simulink model "FCC_2021_JEVG"  (R2021a)
settings: Solver=VariableStepAuto  StartTime=0.0  StopTime=10  RelTol=1e-3
libraries: fl_lib x8, nesl_utility x3
settings Model: Creator=mluser  LastModifiedBy=user
settings DebuggingCC: UnconnectedInputMsg=none  UnconnectedOutputMsg=none  UnconnectedLineMsg=none
settings ModelReferenceCC: EnableRefExpFcnMdlSchedulingChecks=off
settings RTWCC: Description=Generic Real-Time Target  DLArmComputeVersion=20.02.1

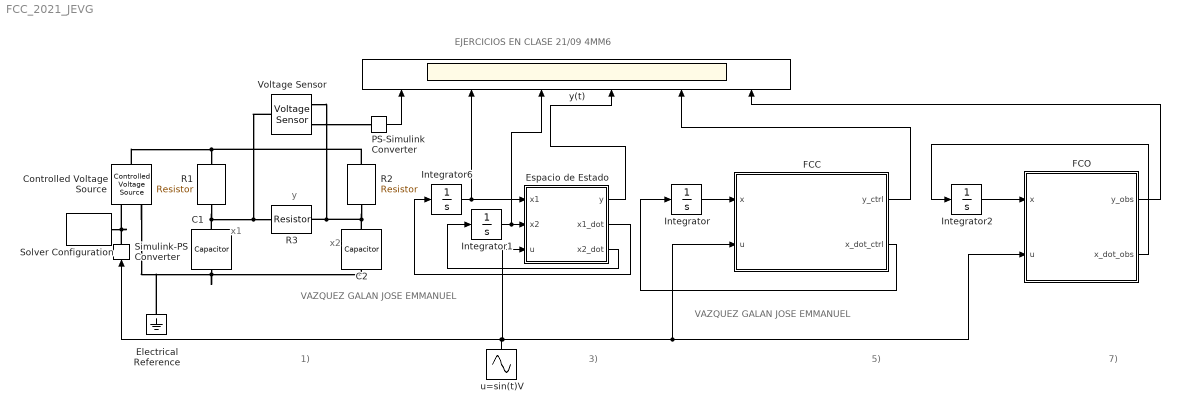
== system FCC_2021_JEVG ==
  note: 1)
  note: EJERCICIOS EN CLASE 21/09 4MM6
  note: VAZQUEZ GALAN JOSE EMMANUEL
  note: y
  note: x1
  note: x2
  note: 3)
  note: 5)
  note: VAZQUEZ GALAN JOSE EMMANUEL
  note: 7)
  C1 : fl_lib/Electrical/Electrical Elements/Capacitor  c=1 F  r=1e-6 Ohm  g=0 1/Ohm  i_specify=off  i_priority=None  i=0 A  i_nominal_specify=off  i_nominal_unit=A  i_nominal_value=1  v_specify=off  v_priority=None  v=0 V  v_nominal_specify=off  v_nominal_unit=V  v_nominal_value=1  vc_specify=on  vc_priority=High  vc=10 V  vc_nominal_specify=off  vc_nominal_unit=V  vc_nominal_value=1
  C2 : fl_lib/Electrical/Electrical Elements/Capacitor  c=2 F  r=1e-6 Ohm  g=0 1/Ohm  i_specify=off  i_priority=None  i=0 A  i_nominal_specify=off  i_nominal_unit=A  i_nominal_value=1  v_specify=off  v_priority=None  v=0 V  v_nominal_specify=off  v_nominal_unit=V  v_nominal_value=1  vc_specify=on  vc_priority=High  vc=5 V  vc_nominal_specify=off  vc_nominal_unit=V  vc_nominal_value=1
  Controlled Voltage Source : fl_lib/Electrical/Electrical Sources/Controlled Voltage Source
  Electrical Reference : fl_lib/Electrical/Electrical Elements/Electrical Reference
  Espacio de Estado : MATLAB Function  TreatAsAtomicUnit=on
  "FCC " : MATLAB Function  TreatAsAtomicUnit=on
  FCO : MATLAB Function  TreatAsAtomicUnit=on
  Integrator : Integrator  InitialCondition=[6.6667 -6.6667 ; -2.2222 8.888889]* [10;5];
  Integrator1 : Integrator  InitialCondition=5
  Integrator2 : Integrator  InitialCondition=[0.05 -0.2; 1 -1]*[10;5];
  Integrator6 : Integrator  InitialCondition=10
  PS-Simulink Converter : nesl_utility/PS-Simulink Converter  PhysicalDomain=network_engine_domain  SubClassName=ps_output  LeftPortType=input  RightPortType=output  PseudoPeriodic=off  Frequencies=[]  Unit=inherit  AffineConversion=off
      settings: SourceProductBaseCode=PW,SS
  R1 : fl_lib/Electrical/Electrical Elements/Resistor  R=5 Ohm  i_specify=off  i_priority=None  i=0 A  i_nominal_specify=off  i_nominal_unit=A  i_nominal_value=1  v_specify=off  v_priority=None  v=0 V  v_nominal_specify=off  v_nominal_unit=V  v_nominal_value=1
  R2 : fl_lib/Electrical/Electrical Elements/Resistor  R=10 Ohm  i_specify=off  i_priority=None  i=0 A  i_nominal_specify=off  i_nominal_unit=A  i_nominal_value=1  v_specify=off  v_priority=None  v=0 V  v_nominal_specify=off  v_nominal_unit=V  v_nominal_value=1
  R3 : fl_lib/Electrical/Electrical Elements/Resistor  R=1 Ohm  i_specify=off  i_priority=None  i=0 A  i_nominal_specify=off  i_nominal_unit=A  i_nominal_value=1  v_specify=off  v_priority=None  v=0 V  v_nominal_specify=off  v_nominal_unit=V  v_nominal_value=1
  Simulink-PS Converter : nesl_utility/Simulink-PS Converter  PhysicalDomain=network_engine_domain  SubClassName=ps_input  LeftPortType=input  RightPortType=output  PseudoPeriodic=off  Frequencies=[]  NoiseDistribution=none  NoiseParameters=[]  Unit=1  AffineConversion=off  FilteringAndDerivatives=provide  SimscapeFilterOrder=1  InputFilterTimeConstant=0.001  UdotUserProvided=0
      settings: SourceProductBaseCode=PW,SS
  Solver Configuration : nesl_utility/Solver Configuration  PhysicalDomain=network_engine_domain  SubClassName=solver  LeftPortType=input  RightPortType=generic  Tones=[]  Harmonics=[]  SimulateNoise=off  Profile=off  UseLocalSampling=off  EnableSwitchedLinearOptims=on  FrequencyDomain=off  UseCCode=off  RelTol=0.001  AbsTol=0.001  MinStep=1e-09  ToWorkspace=off  RevertToSquareIcSolve=off  NumHomotopyIterations=100  PhasorMode=off  PhasorModeNumHarmonics=1  DoDC=off  ResidualTolerance=1e-09  UseLocalSolver=off  LocalSolverChoice=NE_BACKWARD_EULER_ADVANCER  LocalSolverSampleTime=0.001  DoFixedCost=off  MaxNonlinIter=3  MaxModeIter=2  ComputeImpulses=off  ImpulseIterations=2  LinearAlgebra=auto  EquationFormulation=NE_TIME_EF  DelaysMemoryBudget=1024  AutomaticFiltering=on  FilteringTimeConstant=0.001  PartitionStorageMethod=AS_NEEDED  PartitionMemoryBudget=1024  PartitionMethod=ROBUST
      settings: SourceProductBaseCode=PW,SS
  Voltage Sensor : fl_lib/Electrical/Electrical Sensors/Voltage Sensor
  u=sin⁡(t)V : Sin  Amplitude=10  SampleTime=0
  y(t) : Scope  NumInputPorts=6
  wires:
  u=sin⁡(t)V/1 -> FCO/2(u), "FCC "/2(u), Espacio de Estado/3(u), Simulink-PS Converter/1
  PS-Simulink Converter/1 -> y(t)/1
  Integrator1/1 -> y(t)/3, Espacio de Estado/2(x2)
  Integrator6/1 -> Espacio de Estado/1(x1), y(t)/2
  Espacio de Estado/2(x1_dot) -> Integrator6/1
  Espacio de Estado/1(y) -> y(t)/4
  Espacio de Estado/3(x2_dot) -> Integrator1/1
  Integrator/1 -> "FCC "/1(x)
  "FCC "/2(x_dot_ctrl) -> Integrator/1
  "FCC "/1(y_ctrl) -> y(t)/5
  Integrator2/1 -> FCO/1(x)
  FCO/2(x_dot_obs) -> Integrator2/1
  FCO/1(y_obs) -> y(t)/6
  connections:
  R1/RConn1 -- C1/LConn1 -- Voltage Sensor/LConn1 -- R3/LConn1
  R2/RConn1 -- C2/LConn1 -- Voltage Sensor/RConn2 -- R3/RConn1
  C1/RConn1 -- Electrical Reference/LConn1 -- Controlled Voltage Source/RConn2 -- C2/RConn1
  R2/LConn1 -- Controlled Voltage Source/LConn1 -- R1/LConn1
  Simulink-PS Converter/RConn1 -- Solver Configuration/RConn1 -- Controlled Voltage Source/RConn1
  Voltage Sensor/RConn1 -- PS-Simulink Converter/LConn1

== matlab function FCC_2021_JEVG/FCO ==
  data: y_obs output; x input; u input; x_dot_obs output
function [y_obs, x_dot_obs] = sistema_ss_observable(x, u)
    
    % Definición de los parámetros del sistema
    R1 = 5;    % ohms
    R2 = 10;   % ohms
    R3 = 1;    % ohms
    C1 = 1;    % Farads
    C2 = 2;    % Farads

    % Matrices A, B y C originales
    A = [-((C1 * R3 + C1 * R1) / (C1^2 * R1 * R3)), 1/(C1 * R3);
         1/(C2 * R3), -((C2 * R2 + C2 * R3) / (C2^2 * R2 * R3))];
    B = [1/(C1 * R1); 1/(C2 * R2)];
    C = [1, -1];

    a1 = 17/10; % Coeficiente de s^1
    a2 = 3/20;  % Coeficiente de s^0
    
    % Cálculo de S_inv usando a1 y a2
    S_inv = [a1 1; 1 0] * [C; C*A];
    S = (S_inv)^(-1);
    
    % Transformación a forma canónica observable
    A_obs = [0 -0.16; 1 -1.75] 
    B_obs = [0 ; 0.15]     
    C_obs = [0 1] 
    
    % Calcula la derivada de estado y la salida para el sistema observable
    x_dot_obs = A_obs * x + B_obs * u;
    y_obs = C_obs * x;
    
end

== matlab function FCC_2021_JEVG/Espacio de Estado ==
  data: y output; x1 input; x2 input; u input; x1_dot output; x2_dot output
function [y, x1_dot, x2_dot] = sistema_ss(x1, x2, u)

% Definición de los parámetros del sistema
R1 = 5;    % ohms
R2 = 10;   % ohms
R3 = 1;    % ohms
C1 = 1;    % Farads
C2 = 2;    % Farads

% Definición de las matrices A, B y C
A = [-((C1 * R3 + C1 * R1) / (C1^2 * R1 * R3)), 1/(C1 * R3);
      1/(C2 * R3), -((C2 * R2 + C2 * R3) / (C2^2 * R2 * R3))];

B = [1/(C1 * R1); 
     1/(C2 * R2)];

C = [1, -1];

% Calcula la derivada de estado y la salida
x_dot = A * [x1; x2] + B * u;
x1_dot = x_dot(1);
x2_dot = x_dot(2);

y = C * [x1; x2];

end

== matlab function FCC_2021_JEVG/FCC  ==
  data: x input; u input; y_ctrl output; x_dot_ctrl output
function [y_ctrl, x_dot_ctrl] = sistema_ss_controlable(x, u)

    % Definición de los parámetros del sistema
    R1 = 5;    % ohms
    R2 = 10;   % ohms
    R3 = 1;    % ohms
    C1 = 1;    % Farads
    C2 = 2;    % Farads

    % Matrices A, B y C originales
    A = [-((C1 * R3 + C1 * R1) / (C1^2 * R1 * R3)), 1/(C1 * R3);
         1/(C2 * R3), -((C2 * R2 + C2 * R3) / (C2^2 * R2 * R3))];
    B = [1/(C1 * R1); 1/(C2 * R2)];
    C = [1, -1];

    a1 = 17/10; % Coeficiente de s^1
    a2 = 3/20; % Coeficiente de s^0

    % Cálculo de Pinv usando a1 y a2
    Pinv = [B A*B] * [1 a1; 0 1];
    P = inv(Pinv); 

    % Transformación a forma canónica controlable
    % Transformación a forma canónica controlable
    At = [-1.7, -0.15; 1,0];
    Bt = [1; 0];
    Ct = [0.15, 0]

    % Calcula la derivada de estado y la salida para el sistema controlable
    x_dot_ctrl = At * x + Bt * u;
    y_ctrl = Ct * x;

end
